simulink model "ex_2"  (R2017b)
settings: Solver=VariableStepAuto  StartTime=0.0  StopTime=10.0  RelTol=1e-3
undefined symbols (not defined in the file or in its folder): fdesignblkfcn, gcbh
libraries: simulink x1, dspfdesign x1
settings Model: Creator=tongbohan  LastModifiedBy=tongbohan

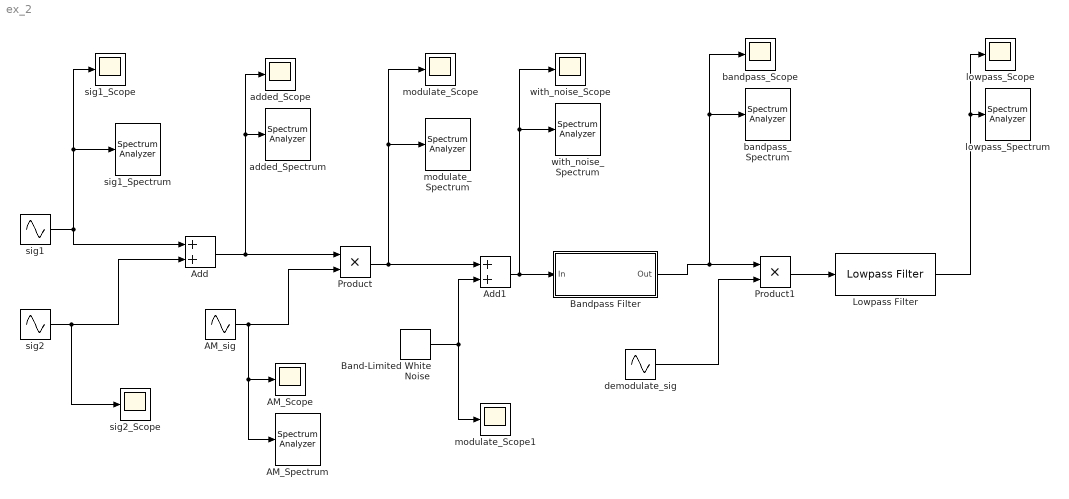
== system ex_2 ==
  AM_Scope : Scope
  AM_Spectrum : SpectrumAnalyzer
  AM_sig : Sin  Amplitude=100  Frequency=500  SampleTime=1/2000
  Add : Sum
  Add1 : Sum
  Band-Limited White Noise : simulink/Sources/Band-Limited White Noise  Cov=[0.1]  Ts=0.1  seed=[23341]
  Bandpass Filter : Subsystem  DialogController=fdesignblkfcn  InitFcn=fdesignblkfcn(gcbh, {'InitFcn'});  mask(Bandpass Filter){}
      mask help: Design a bandpass filter
      settings: CopyFcn=fdesignblkfcn(gcbh, {'CopyFcn'});
      mask Help: helpview(mapfilelocation('dsp'), 'dspbandpassfilter');
      mask Display: disp('Bandpass');
  Lowpass Filter : dspfdesign/Lowpass Filter  FilterType=IIR  DesignForMinimumOrder=on  FilterOrder=50  PassbandFrequency=14  StopbandFrequency=18  PassbandRipple=1  StopbandAttenuation=170  InheritSampleRate=off  SampleRate=2000  SimulateUsing=Interpreted execution  roundingMode=Floor  coeffsDataTypeStr=fixdt(1,16)
  Product : Product
  Product1 : Product
  added_Scope : Scope
  added_Spectrum : SpectrumAnalyzer
  bandpass_Scope : Scope
  bandpass_Spectrum : SpectrumAnalyzer
  demodulate_sig : Sin  Amplitude=100  Frequency=500  SampleTime=1/2000
  lowpass_Scope : Scope
  lowpass_Spectrum : SpectrumAnalyzer
  modulate_Scope : Scope
  modulate_Scope1 : Scope
  modulate_Spectrum : SpectrumAnalyzer
  sig1 : Sin  Frequency=50  SampleTime=1/2000
  sig1_Scope : Scope
  sig1_Spectrum : SpectrumAnalyzer
  sig2 : Sin  Amplitude=2  Frequency=0  Phase=90  SampleTime=1/2000
  sig2_Scope : Scope
  with_noise_Scope : Scope
  with_noise_Spectrum : SpectrumAnalyzer
  wires:
  sig1/1 -> Add/1, sig1_Spectrum/1, sig1_Scope/1
  sig2/1 -> sig2_Scope/1, Add/2
  AM_sig/1 -> AM_Scope/1, AM_Spectrum/1, Product/2
  Add/1 -> added_Spectrum/1, added_Scope/1, Product/1
  demodulate_sig/1 -> Product1/2
  Product1/1 -> Lowpass Filter/1
  Lowpass Filter/1 -> lowpass_Scope/1, lowpass_Spectrum/1
  Product/1 -> Add1/1, modulate_Scope/1, modulate_Spectrum/1
  Band-Limited White Noise/1 -> modulate_Scope1/1, Add1/2
  Add1/1 -> Bandpass Filter/1(In), with_noise_Spectrum/1, with_noise_Scope/1
  Bandpass Filter/1(Out) -> bandpass_Spectrum/1, bandpass_Scope/1, Product1/1

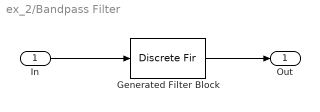
== system ex_2/Bandpass Filter ==
  In : Inport
  Generated Filter Block : DiscreteFir  Tag=BlockMethodSubSystem  Coefficients=[-0.000271528895255182588 0.000352756454276449271 2.69730664487950518e-05 -0.000123272105641871805 -0.000139706643555305475 -7.63370232388889197e-05 1.8833652861051208e-05 0.00011299836784680959 0.000189046779672542598 0.00024241523034914536 0.000275474344072578316 0.000293320610436316475 0.000300164189458403672 0.000298339804875837316 0.000287716360195111836 0.000266872148787799547 0.000233586404850738853 0.000186252311743212115 0.000124016611562246252 4.76327375551396711e-05 -4.10104459610567882e-05 -0.000138482490898435149 -0.000240610129074697642 -0.000342210041513745693 -0.000437984878077861981 -0.000522225263130854638 -0.000589735800964473868 -0.000635468902919660516 -0.000655487977906242807 -0.000646508017698320197 -0.000606873417875030438 -0.000535950262028780282 -0.000435080810348210695 -0.00030674744289095466 -0.000155479163532881552 1.32872050563002886e-05 0.000192312745608359137 0.000374054452036855071 0.000549677019523377424 0.000710981967438324507 0.000849074692989385395 0.000956929558230999212 0.00102719533394657575 0.00105585987319681534 0.00103857853861990613 0.000975303213385315883 0.000866597002312649947 0.000715300966421360349 0.000528578318102551495 0.000311554200158269264 7.50884718782264722e-05 -0.000171002763771957856 -0.00041623473333337284 -0.000649061807354267897 -0.000857954031545728993 -0.00103391907804199421 -0.00116813409139179358 -0.00125355928226200328 -0.00128571564892620595 -0.00126327122427809637 -0.00118649070921511427 -0.00105842843960959887 -0.000884831810131566851 -0.00067406229397103687 -0.000435548437588089527 -0.000180136254550205687 8.04660772613336004e-05 0.000333951063508870934 0.000568941841103041274 0.000775119902275384401 0.000943771609748016551 0.00106770941619525363 0.00114228240468556902 0.00116541632814188526 0.00113788064765677909 0.00106259730182732873 0.000944797644991662118 0.000791582346234088585 0.000611925362978252741 0.000415693053589648255 0.000213223539403330909 1.44639416962390083e-05 -0.000171097050492885364 -0.000335152971253573897 -0.000470766458145810581 -0.000573199035216194475 -0.000639687014006543107 -0.000669981318345102823 -0.000665343887426568092 -0.000629592133182723312 -0.000567267846251031803 -0.000485373864845441074 -0.000390607591605078304 -0.00029080229193376839 -0.000193089250066319967 -0.000103760121573345001 -2.85726379259350143e-05 2.84693196665156274e-05 6.4974815853931144e-05 7.9951993891571048e-05 7.46929083438321807e-05 5.19566313510047085e-05 1.56310000078250292e-05 -2.92102544437285005e-05 -7.67187021359560454e-05 -0.000121134092634507957 -0.000156663829625797396 -0.000178090945735003139 -0.000181408956596321234 -0.000164168853115362253 -0.000125237609298303428 -6.52435518631895985e-05 1.34652888042539448e-05 0.000106984295848897509 0.000210273694526170649 0.000317069668264341443 0.000420477694360330077 0.000513471902529992409 0.000589556690183695221 0.000642835048476739029 0.000668604088690838688 0.000663619045979568409 0.000626517247218576819 0.000557629619126857445 0.000459266280560770746 0.000335508202639311296 0.000192215675813788695 3.62789944839330634e-05 -0.000124505434823308505 -0.000282127710277126683 -0.000428405161254296566 -0.000555959433679194953 -0.000658256577237697495 -0.000730382201744303569 -0.000768948513914267462 -0.000772510635358520477 -0.000741784693306943321 -0.000679145838229300129 -0.000589045902542378896 -0.000476921657820315631 -0.000349595345086025201 -0.000214523064113330522 -7.92547823632218119e-05 4.87878968364037578e-05 0.000163075898237571366 0.000258275429806492022 0.000330313112130207294 0.000376963713049421173 0.000397805222830070737 0.000394035702467749325 0.000368528703307764911 0.000325519402983407411 0.000270172162092939224 0.00020841527329710862 0.000146439509830661546 9.00300690571418987e-05 4.42658526669155867e-05 1.32322294263816366e-05 -3.96685490294091784e-07 4.45637992854947053e-06 2.73074062881172255e-05 6.60384391044281725e-05 0.000117008970159100911 0.000175430755898947188 ...(+27649 chars)]  InputProcessing=Columns as channels (frame based)
  Out : Outport
  wires:
  In/1 -> Generated Filter Block/1
  Generated Filter Block/1 -> Out/1
